simulink model "Diagramas_de_bloques"  (R2018a)
settings: Solver=VariableStepAuto  StartTime=0.0  StopTime=10  RelTol=1e-3
libraries: simulink x1
settings Model: Creator=Paulo  LastModifiedBy=Paulo

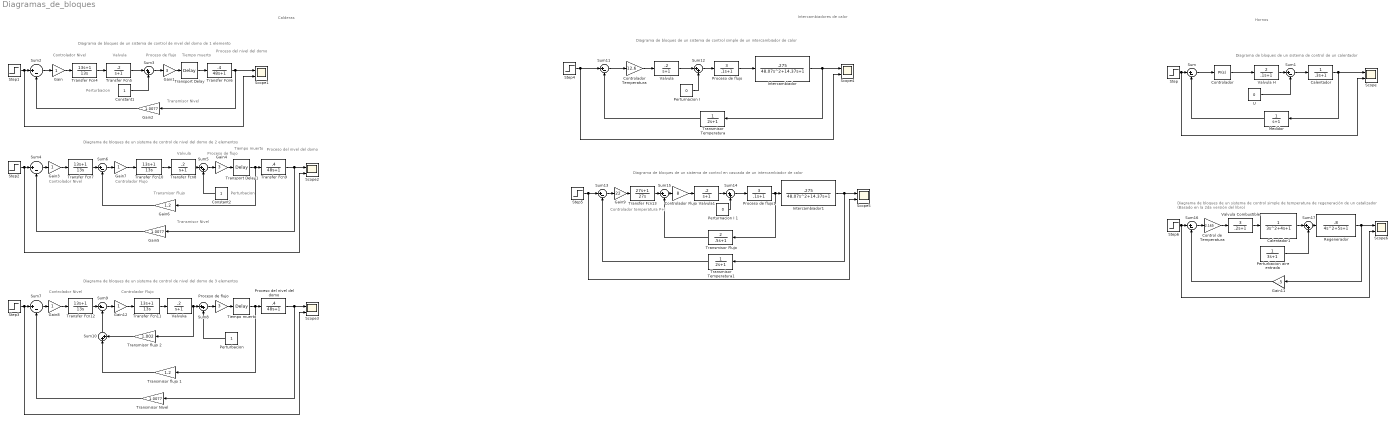
== system Diagramas_de_bloques ==
  note: Diagrama de bloques de un sistema de control de un calentador
  note: Controlador temperatura
      | P+I
  note: Transmisor Nivel
  note: Perturbacion
  note: Proceso del nivel
      |  del domo
  note: Tiempo muerto
  note: Proceso de flujo
  note: Valvula
  note: Diagrama de bloques de un sistema de control de nivel del domo de 1 elemento
  note: Calderas
  note: Intercambiadores de calor
  note: Hornos
  note: Diagrama de bloques de un sistema de control de nivel del domo de 2 elementos
  note: Controlador Flujo
  note: Controlador Nivel
  note: Valvula
  note: Proceso de
      |  flujo
  note: Tiempo muerto
  note: Proceso del nivel
      | del domo
  note: Perturbacion
  note: Transmisor Nivel
  note: Controlador Nivel
  note: Transmisor Flujo
  note: Controlador Nivel
  note: Controlador Flujo
  note: Diagrama de bloques de un sistema de control de nivel del domo de 3 elementos
  note: Diagrama de bloques de un sistema de control simple de un intercambiador de calor
  note: Diagrama de bloques de un sistema de control en cascada de un intercambiador de calor
  note: Diagrama de bloques de un sistema de control simple de temperatura de regeneración de un catalizador
      | (Basado en la 2da versión del libro)
  Calentador : TransferFcn  Denominator=[.3 1]
  Calentador1 : TransferFcn  Denominator=[3 4 1]
  Constant1 : Constant
  Constant2 : Constant
  Control de Temperatura : Gain  Gain=2.165
  Controlador : simulink/Continuous/PID Controller  Controller=PI  TimeDomain=Continuous-time  SampleTime=-1  IntegratorMethod=Forward Euler  FilterMethod=Forward Euler  Form=Ideal  UseFilter=on  ControllerParametersSource=internal  P=2.2  I=1/.75  D=0  N=100  InitialConditionSource=internal  InitialConditionForIntegrator=0  InitialConditionForFilter=0  ExternalReset=none  LimitOutput=off  UpperSaturationLimit=inf  LowerSaturationLimit=-inf  LinearizeAsGain=on  AntiWindupMode=none  Kb=1  TrackingMode=off  Kt=1  PParamMin=[]  PParamMax=[]  IParamMin=[]  IParamMax=[]  DParamMin=[]  DParamMax=[]  NParamMin=[]  NParamMax=[]  KbParamMin=[]  KbParamMax=[]  KtParamMin=[]  KtParamMax=[]  POutMin=[]  POutMax=[]  IOutMin=[]  IOutMax=[]  DOutMin=[]  DOutMax=[]  NOutMin=[]  NOutMax=[]  KbOutMin=[]  KbOutMax=[]  KtOutMin=[]  KtOutMax=[]  IntegratorOutMin=[]  IntegratorOutMax=[]  FilterOutMin=[]  FilterOutMax=[]  SumOutMin=[]  SumOutMax=[]  SumI1OutMin=[]  SumI1OutMax=[]  SumI2OutMin=[]  SumI2OutMax=[]  SumI3OutMin=[]  SumI3OutMax=[]  SumDOutMin=[]  SumDOutMax=[]  SaturationOutMin=[]  SaturationOutMax=[]  IntegratorContinuousStateAttributes=''  IntegratorStateMustResolveToSignalObject=off  IntegratorRTWStateStorageClass=Auto  FilterContinuousStateAttributes=''  FilterStateMustResolveToSignalObject=off  FilterRTWStateStorageClass=Auto  DifferentiatorICPrevScaledInput=0  DifferentiatorOutMin=[]  DifferentiatorOutMax=[]  FilterDiffOutCoefMin=[]  FilterDiffOutCoefMax=[]  SumDenOutMin=[]  SumDenOutMax=[]  SumNumOutMin=[]  SumNumOutMax=[]  ReciprocalOutMin=[]  ReciprocalOutMax=[]  DivideOutMin=[]  DivideOutMax=[]  TunerSelectOption=Transfer Function Based (PID Tuner App)
  Controlador Flujo : Gain  Gain=8
  Controlador Temperatura : Gain  Gain=12.6
  Gain{,3,7..8,12} (5 alike) : Gain
  Gain1 : Gain  Gain=3
  Gain11 : Gain  Gain=.5
  Gain2 : Gain  Gain=1.0077
  Gain4 : Gain  Gain=3
  Gain5 : Gain  Gain=1.0077
  Gain6 : Gain  Gain=1.2
  Gain9 : Gain  Gain=22
  Intercambiador : TransferFcn  Numerator=[.275]  Denominator=[48.07 14.37 1]
  Intercambiador1 : TransferFcn  Numerator=[.275]  Denominator=[48.07 14.37 1]
  Medidor : TransferFcn  Denominator=[1 1]
  Perturbacion : Constant
  Perturbacion aire entrada : TransferFcn  Denominator=[3 1]
  "Perturnacion I " : Constant  Value=0
  Perturnacion I 1 : Constant  Value=0
  Proceso de flujo : Gain  Gain=3
  Proceso de flujo : TransferFcn  Numerator=[3]  Denominator=[.1 1]
  Proceso de flujo1 : TransferFcn  Numerator=[3]  Denominator=[.1 1]
  Proceso del nivel del domo : TransferFcn  Numerator=[.4]  Denominator=[48 1]
  "Regenerador " : TransferFcn  Numerator=[.8]  Denominator=[4 5 1]
  Scope{,1..6} (7 alike) : Scope  NumInputPorts=2
  Step{,1..6} (7 alike) : Step  Time=0  SampleTime=0
  Sum{,1..2,4,6..7,9,11,13,15..16} (11 alike) : Sum  Inputs=|+-
  Sum{3,5,8,10,12,14,17} (7 alike) : Sum  Inputs=|++
  Tiempo muerto : TransportDelay
  Transfer Fcn{4,7,10..12} (5 alike) : TransferFcn  Numerator=[13 1]  Denominator=[13 0]
  Transfer Fcn13 : TransferFcn  Numerator=[27 1]  Denominator=[27 0]
  Transfer Fcn5 : TransferFcn  Numerator=[.2]  Denominator=[1 1]
  Transfer Fcn6 : TransferFcn  Numerator=[.4]  Denominator=[48 1]
  Transfer Fcn8 : TransferFcn  Numerator=[.2]  Denominator=[1 1]
  Transfer Fcn9 : TransferFcn  Numerator=[.4]  Denominator=[48 1]
  "Transmisor Flujo " : TransferFcn  Numerator=[2]  Denominator=[.5 1]
  Transmisor Nivel : Gain  Gain=1.0077
  Transmisor Temperatura : TransferFcn  Denominator=[2 1]
  Transmisor Temperatura1 : TransferFcn  Denominator=[2 1]
  Transmisor flujo 1 : Gain  Gain=1.2
  Transmisor flujo 2 : Gain  Gain=1.002
  Transport Delay : TransportDelay
  Transport Delay1 : TransportDelay
  U : Constant  Value=0
  Valvuka : TransferFcn  Numerator=[.2]  Denominator=[1 1]
  Valvula : TransferFcn  Numerator=[.2]  Denominator=[1 1]
  Valvula Combustible : TransferFcn  Numerator=[3]  Denominator=[.2 1]
  Valvula H : TransferFcn  Numerator=[2]  Denominator=[.1 1]
  Valvula1 : TransferFcn  Numerator=[.2]  Denominator=[1 1]
  wires:
  Step/1 -> Scope/2, Sum/1
  Valvula H/1 -> Sum1/1
  Sum1/1 -> Calentador/1
  Calentador/1 -> Scope/1, Medidor/1
  U/1 -> Sum1/2
  Medidor/1 -> Sum/2
  Step1/1 -> Scope1/2, Sum2/1
  Sum2/1 -> Gain/1
  Gain/1 -> Transfer Fcn4/1
  Transfer Fcn4/1 -> Transfer Fcn5/1
  Transfer Fcn5/1 -> Sum3/1
  Sum3/1 -> Gain1/1
  Gain1/1 -> Transport Delay/1
  Transport Delay/1 -> Transfer Fcn6/1
  Transfer Fcn6/1 -> Gain2/1, Scope1/1
  Constant1/1 -> Sum3/2
  Gain2/1 -> Sum2/2
  Transport Delay1/1 -> Gain6/1, Transfer Fcn9/1
  Constant2/1 -> Sum5/2
  Gain5/1 -> Sum4/2
  Sum4/1 -> Gain3/1
  Transfer Fcn9/1 -> Gain5/1, Scope2/1
  Gain4/1 -> Transport Delay1/1
  Step2/1 -> Sum4/1, Scope2/2
  Sum5/1 -> Gain4/1
  Gain3/1 -> Transfer Fcn7/1
  Transfer Fcn8/1 -> Sum5/1
  Transfer Fcn7/1 -> Sum6/1
  Gain6/1 -> Sum6/2
  Gain7/1 -> Transfer Fcn10/1
  Sum6/1 -> Gain7/1
  Transfer Fcn10/1 -> Transfer Fcn8/1
  Gain12/1 -> Transfer Fcn11/1
  Transfer Fcn11/1 -> Valvuka/1
  Transfer Fcn12/1 -> Sum9/1
  Sum9/1 -> Gain12/1
  Valvuka/1 -> Transmisor flujo 2/1, Sum8/1
  Sum8/1 -> Proceso de flujo/1
  Gain8/1 -> Transfer Fcn12/1
  Step3/1 -> Sum7/1, Scope3/2
  Transmisor Nivel/1 -> Sum7/2
  Proceso del nivel del domo/1 -> Transmisor Nivel/1, Scope3/1
  Proceso de flujo/1 -> Tiempo muerto/1
  Perturbacion/1 -> Sum8/2
  Tiempo muerto/1 -> Transmisor flujo 1/1, Proceso del nivel del domo/1
  Sum7/1 -> Gain8/1
  Sum10/1 -> Sum9/2
  Transmisor flujo 2/1 -> Sum10/2
  Transmisor flujo 1/1 -> Sum10/1
  Step4/1 -> Scope4/2, Sum11/1
  Sum11/1 -> Controlador Temperatura/1
  Controlador Temperatura/1 -> Valvula/1
  Valvula/1 -> Sum12/1
  "Perturnacion I "/1 -> Sum12/2
  Sum12/1 -> Proceso de flujo/1
  Proceso de flujo/1 -> Intercambiador/1
  Intercambiador/1 -> Transmisor Temperatura/1, Scope4/1
  Transmisor Temperatura/1 -> Sum11/2
  Transmisor Temperatura1/1 -> Sum13/2
  Controlador Flujo/1 -> Valvula1/1
  Perturnacion I 1/1 -> Sum14/2
  Intercambiador1/1 -> Transmisor Temperatura1/1, Scope5/1
  Proceso de flujo1/1 -> "Transmisor Flujo "/1, Intercambiador1/1
  Sum14/1 -> Proceso de flujo1/1
  Valvula1/1 -> Sum14/1
  Step5/1 -> Scope5/2, Sum13/1
  Sum13/1 -> Gain9/1
  Gain9/1 -> Transfer Fcn13/1
  Transfer Fcn13/1 -> Sum15/1
  Sum15/1 -> Controlador Flujo/1
  "Transmisor Flujo "/1 -> Sum15/2
  Gain11/1 -> Sum16/2
  Step6/1 -> Scope6/2, Sum16/1
  Perturbacion aire entrada/1 -> Sum17/2
  Calentador1/1 -> Sum17/1
  Sum16/1 -> Control de Temperatura/1
  Control de Temperatura/1 -> Valvula Combustible/1
  Valvula Combustible/1 -> Calentador1/1
  Sum17/1 -> "Regenerador "/1
  "Regenerador "/1 -> Gain11/1, Scope6/1
  Controlador/1 -> Valvula H/1
  Sum/1 -> Controlador/1
